simulink model "p8sim"  (R2017b)
settings: Solver=VariableStepAuto  StartTime=0.0  StopTime=10.0  RelTol=1e-3
values from neighbouring files (symbols this model uses):
  L = acker(A1',C1',[zo zo zo])    [p10.m]    (also in p8.m)
undefined symbols (not defined in the file or in its folder): A, C
settings Model: Creator=Tomek  LastModifiedBy=Tomek

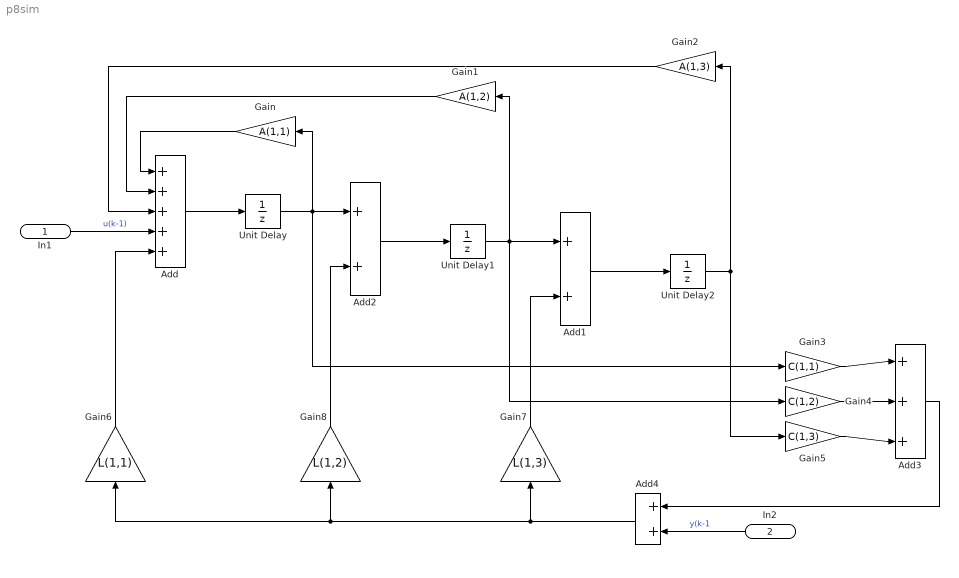
== system p8sim ==
  In1 : Inport
  In2 : Inport  Port=2
  Add : Sum  Inputs=+++++
  Add1 : Sum
  Add2 : Sum
  Add3 : Sum  Inputs=+++
  Add4 : Sum
  Gain : Gain  Gain=A(1,1)
  Gain1 : Gain  Gain=A(1,2)
  Gain2 : Gain  Gain=A(1,3)
  Gain3 : Gain  Gain=C(1,1)
  Gain4 : Gain  Gain=C(1,2)
  Gain5 : Gain  Gain=C(1,3)
  Gain6 : Gain  Gain=L(1,1)
  Gain7 : Gain  Gain=L(1,3)
  Gain8 : Gain  Gain=L(1,2)
  Unit Delay : UnitDelay  SampleTime=-1
  Unit Delay1 : UnitDelay  SampleTime=-1
  Unit Delay2 : UnitDelay  SampleTime=-1
  wires:
  Add/1 -> Unit Delay/1
  Unit Delay/1 -> Gain3/1, Gain/1, Add2/1
  Add2/1 -> Unit Delay1/1
  Unit Delay1/1 -> Gain4/1, Add1/1, Gain1/1
  Add1/1 -> Unit Delay2/1
  Gain/1 -> Add/1
  Gain1/1 -> Add/2
  Gain2/1 -> Add/3
  Unit Delay2/1 -> Gain5/1, Gain2/1
  Gain3/1 -> Add3/1
  Gain4/1 -> Add3/2
  Gain5/1 -> Add3/3
  In1/1 -> Add/4  "u(k-1)"
  Gain6/1 -> Add/5
  Gain8/1 -> Add2/2
  Gain7/1 -> Add1/2
  In2/1 -> Add4/2  "y(k-1"
  Add3/1 -> Add4/1
  Add4/1 -> Gain7/1, Gain8/1, Gain6/1
